simulink model "HybridControllerD2D2"  (R2020b)
settings: Solver=ode8  StartTime=0.0  StopTime=inf  FixedStep=samplePeriod  RelTol=1e-3  AbsTol=1e-6  EnableMultiTasking=on
PreLoadFcn:
  | initializeSimulation;
InitFcn:
  | clear('all');
  | initializeSimulation;
values from neighbouring files (symbols this model uses):
  adaptivegain = diag(10.^[6.03 4.23 1.48 -1.10])    [initializeSimulation.m]
  Area = 0.751    [initializeSimulation.m]
  Be = 95958    [initializeSimulation.m]
  Cl = 5.89e-6    (= 5.89e-06)    [initializeSimulation.m]
  coef = 1.0    (= 1)    [initializeSimulation.m]
  damperB = 0    [initializeSimulation.m]
  damperCanon = 1    [initializeSimulation.m]
  Derivadas = [u;dudt;dudt2;dudt3]    [initializeSimulation.m]
  fir_coef = length(dAMB_i)    [initializeSimulation.m]
  forceCanon = 1    [initializeSimulation.m]
  forgfact = 1    [initializeSimulation.m]
  frictionB = 0    [initializeSimulation.m]
  Gsnsr_DT = 1    [initializeSimulation.m]
  Gsnsr_FT = 1    [initializeSimulation.m]
  Kc = 1.36e-5    (= 1.36e-05)    [initializeSimulation.m]
  Kp = 3.0    (= 3)    [initializeSimulation.m]
  Kq = 23.01    [initializeSimulation.m]
  kv = 1    [initializeSimulation.m]
  lengthCanon = 1    [initializeSimulation.m]
  max_amb = [amb0max,amb1max,amb2max,amb3max]*1e15    [initializeSimulation.m]
  maxDisplB = (stroke2B + endLength2B) * lengthCanon    (= 42)    [initializeSimulation.m]
  maxVelocB = (maxFlowB * flowCanon / (area1B * areaCanon)) / velocCanon    [initializeSimulation.m]
  me = 0.023/1000    (= 2.3e-05)    [initializeSimulation.m]
  min_amb = [amb0min,amb1min,amb2min,amb3min]    [initializeSimulation.m]
  minDisplB = -(stroke1B + endLength1B) * lengthCanon    (= -42)    [initializeSimulation.m]
  minVelocB = -(maxFlowB * flowCanon / (area2B * areaCanon)) / velocCanon    [initializeSimulation.m]
  MRC = [2 0.05 0.001]    [initializeSimulation.m]
  Nl = floor(tl*sample_rate)    [initializeSimulation.m]
  P_corr_i = eye(4)*1e10    [initializeSimulation.m]
  P_range = [0.7 1.30 ... (first row only)    [initializeSimulation.m]
  samplePeriod = 0.5/1024    (= 0.00048828125)    [initializeSimulation.m]
  sat_limit_lower = -3.8    [initializeSimulation.m]
  sat_limit_upper = +3.8    (= 3.8)    [initializeSimulation.m]
  Seed_snr = rng(seed)    [initializeSimulation.m]
  SN = 16    [initializeSimulation.m]
  staticForceB = 0    [initializeSimulation.m]
  tauv = 0.00332    [initializeSimulation.m]
  velocCanon = 1    [initializeSimulation.m]
  Vt = 48.66    [initializeSimulation.m]
  yieldDisplB = 0.1    [initializeSimulation.m]
  Zden = ztag.Denominator{1}    [initializeSimulation.m]
  Znum = ztag.Numerator{1}    [initializeSimulation.m]
undefined symbols (not defined in the file or in its folder): denfilter, DiscIntNeverNeededParam, HybridCtrlParameters, numfilter, Par, Threshold
libraries: simulink x17, sldrtlib x1, dsparch4 x1
(part 2 of 2)

== matlab function HybridControllerD2D2/model/ATS compensator/calculate optimal coefficients ==
  data: threshold input; par input; p_range input; MRC input; X1 input; apar output; X2 input; X3 input; Y input; dm input; prev_par input; triggeri input
function apar = fcn(threshold,par,p_range,MRC,X1,X2,X3,Y,dm,prev_par,triggeri)
%#codegen
%triggero=triggeri;
apar = [par; triggeri];

if( abs( dm ) > threshold || apar(4) )
    apar(4)=1;
    
    X = [X1 X2 X3];       
    
    temp=X\Y; 
    
    apar(1:3)=temp;
    
    if( isnan( apar(1) ) + isnan( apar(2) ) + isnan( apar(3) ) )
        apar=[par; triggeri];
    end
    
    
    % maximum change of rate
    if( abs(apar(1)-prev_par(1)) > MRC(1) )
        apar(1) = prev_par(1) + sign(apar(1)-prev_par(1))*MRC(1);
    end
    if( abs(apar(2)-prev_par(2)) > MRC(2) )
        apar(2) = prev_par(2) + sign(apar(2)-prev_par(2))*MRC(2);
    end
    if( abs(apar(3)-prev_par(3)) > MRC(3) )
        apar(3) = prev_par(3) + sign(apar(3)-prev_par(3))*MRC(3);
    end
    
    % limit of coefficients
    if( apar(1) < p_range(1,1) )
        apar(1) = p_range(1,1);
    end
    
    if( apar(1) > p_range(1,2) )
        apar(1) = p_range(1,2);
    end
    
    if( apar(2) < p_range(2,1) )
        apar(2) = p_range(2,1);
    end
    
    if( apar(2) > p_range(2,2) )
        apar(2) = p_range(2,2);
    end
    
    if( apar(3) < p_range(3,1) )
        apar(3) = p_range(3,1);
    end
    
    if( apar(3) > p_range(3,2) )
        apar(3) = p_range(3,2);
    end    
    
end
